simulink model "SF051A_SnsrOffsLrng"  (R2013b)
settings: Solver=FixedStepDiscrete  SolverMode=SingleTasking  StartTime=0.0  StopTime=1  FixedStep=0.002  RelTol=1e-3
values from neighbouring files (symbols this model uses):
  ARCHGLBPRM_10MILLISEC_SEC_F32 = DataDict.Constant    [SF051A_SnsrOffsLrng_DataDict.m]
  ARCHGLBPRM_2MILLISEC_SEC_F32 = DataDict.Constant    [SF051A_SnsrOffsLrng_DataDict.m]
  ARCHGLBPRM_2PI_ULS_F32 = DataDict.Constant    [SF051A_SnsrOffsLrng_DataDict.m]
  ARCHGLBPRM_FLOATZEROTHD_ULS_F32 = DataDict.Constant    [SF051A_SnsrOffsLrng_DataDict.m]
  ARCHGLBPRM_PIOVER180_ULS_F32 = DataDict.Constant    [SF051A_SnsrOffsLrng_DataDict.m]
  CNV100MICROSECTOSEC_SECPERCNT_F32 = DataDict.Constant    [SF051A_SnsrOffsLrng_DataDict.m]
  COVRAMTRXNIT_ULS_F32 = DataDict.Constant    [SF051A_SnsrOffsLrng_DataDict.m]
  HWAGHILIM_HWDEG_F32 = DataDict.Constant    [SF051A_SnsrOffsLrng_DataDict.m]
  HWAUTHYTHD_ULS_F32 = DataDict.Constant    [SF051A_SnsrOffsLrng_DataDict.m]
  HWTQLRNGSTSLRND_CNT_U08 = DataDict.Constant    [SF051A_SnsrOffsLrng_DataDict.m]
  HWTQLRNGSTSNEGOFFS_CNT_U08 = DataDict.Constant    [SF051A_SnsrOffsLrng_DataDict.m]
  HWTQLRNGSTSNOTLRND_CNT_U08 = DataDict.Constant    [SF051A_SnsrOffsLrng_DataDict.m]
  HWTQLRNGSTSPOSOFFS_CNT_U08 = DataDict.Constant    [SF051A_SnsrOffsLrng_DataDict.m]
  HWTQLRNGSTSZEROOFFS_CNT_U08 = DataDict.Constant    [SF051A_SnsrOffsLrng_DataDict.m]
  IDYMTRX_ULS_F32 = DataDict.Constant    [SF051A_SnsrOffsLrng_DataDict.m]
  IVS10MS_ULSPERSEC_F32 = DataDict.Constant    [SF051A_SnsrOffsLrng_DataDict.m]
  LRNGFILTICON_ULS_F32 = DataDict.Constant    [SF051A_SnsrOffsLrng_DataDict.m]
  ONE_ULS_F32 = DataDict.Constant    [SF051A_SnsrOffsLrng_DataDict.m]
  SnsrOffsLrnd = DataDict.NVM    [SF051A_SnsrOffsLrng_DataDict.m]
  SnsrOffsLrngFctEna = DataDict.Calibration    [SF051A_SnsrOffsLrng_DataDict.m]
  SnsrOffsLrngHwAgLrngDrvgDstThd = DataDict.Calibration    [SF051A_SnsrOffsLrng_DataDict.m]
  SnsrOffsLrngHwAgLrngEna = DataDict.Calibration    [SF051A_SnsrOffsLrng_DataDict.m]
  SnsrOffsLrngHwAgLrngHwVelThd = DataDict.Calibration    [SF051A_SnsrOffsLrng_DataDict.m]
  SnsrOffsLrngHwAgLrngSysTqThd = DataDict.Calibration    [SF051A_SnsrOffsLrng_DataDict.m]
  SnsrOffsLrngHwAgLrngSysTqThdMed = DataDict.Calibration    [SF051A_SnsrOffsLrng_DataDict.m]
  SnsrOffsLrngHwAgLrngSysTqThdTrustd = DataDict.Calibration    [SF051A_SnsrOffsLrng_DataDict.m]
  SnsrOffsLrngHwAgLrngSysTqThdWide = DataDict.Calibration    [SF051A_SnsrOffsLrng_DataDict.m]
  SnsrOffsLrngHwAgLrngTi = DataDict.Calibration    [SF051A_SnsrOffsLrng_DataDict.m]
  SnsrOffsLrngHwAgLrngVehSpdThd = DataDict.Calibration    [SF051A_SnsrOffsLrng_DataDict.m]
  SnsrOffsLrngHwAgLrngYawOffsDbnd = DataDict.Calibration    [SF051A_SnsrOffsLrng_DataDict.m]
  SnsrOffsLrngHwAgLrngYawRateThd = DataDict.Calibration    [SF051A_SnsrOffsLrng_DataDict.m]
  SnsrOffsLrngHwAgOffsLim = DataDict.Calibration    [SF051A_SnsrOffsLrng_DataDict.m]
  SnsrOffsLrngHwTqLrngEna = DataDict.Calibration    [SF051A_SnsrOffsLrng_DataDict.m]
  SnsrOffsLrngHwTqLrngEnaTiThd = DataDict.Calibration    [SF051A_SnsrOffsLrng_DataDict.m]
  SnsrOffsLrngHwTqLrngHwAgDbnd = DataDict.Calibration    [SF051A_SnsrOffsLrng_DataDict.m]
  SnsrOffsLrngHwTqLrngHwAgThd = DataDict.Calibration    [SF051A_SnsrOffsLrng_DataDict.m]
  SnsrOffsLrngHwTqLrngHwTqThd = DataDict.Calibration    [SF051A_SnsrOffsLrng_DataDict.m]
  SnsrOffsLrngHwTqLrngHwTqZeroOffsThd = DataDict.Calibration    [SF051A_SnsrOffsLrng_DataDict.m]
  SnsrOffsLrngHwTqLrngHwVelThd = DataDict.Calibration    [SF051A_SnsrOffsLrng_DataDict.m]
  SnsrOffsLrngHwTqLrngMeasTi = DataDict.Calibration    [SF051A_SnsrOffsLrng_DataDict.m]
  SnsrOffsLrngHwTqLrngMeasTiScar = DataDict.Calibration    [SF051A_SnsrOffsLrng_DataDict.m]
  SnsrOffsLrngHwTqLrngSampleImbThd1 = DataDict.Calibration    [SF051A_SnsrOffsLrng_DataDict.m]
  SnsrOffsLrngHwTqLrngSampleImbThd2 = DataDict.Calibration    [SF051A_SnsrOffsLrng_DataDict.m]
  SnsrOffsLrngHwTqLrngSampleThd1 = DataDict.Calibration    [SF051A_SnsrOffsLrng_DataDict.m]
  SnsrOffsLrngHwTqLrngSampleThd2 = DataDict.Calibration    [SF051A_SnsrOffsLrng_DataDict.m]
  SnsrOffsLrngHwTqLrngTiWghtCoeff = DataDict.Calibration    [SF051A_SnsrOffsLrng_DataDict.m]
  SnsrOffsLrngHwTqLrngVehSpdThd = DataDict.Calibration    [SF051A_SnsrOffsLrng_DataDict.m]
  SnsrOffsLrngHwTqOffsLim = DataDict.Calibration    [SF051A_SnsrOffsLrng_DataDict.m]
  SnsrOffsLrngSampleCntForHwTqLrngRst = DataDict.Calibration    [SF051A_SnsrOffsLrng_DataDict.m]
  SnsrOffsLrngTqInpDetnPwrEstimnThd = DataDict.Calibration    [SF051A_SnsrOffsLrng_DataDict.m]
  SnsrOffsLrngTqInpDetnSinGenrAmp = DataDict.Calibration    [SF051A_SnsrOffsLrng_DataDict.m]
  SnsrOffsLrngTqInpDetnSinGenrFrq = DataDict.Calibration    [SF051A_SnsrOffsLrng_DataDict.m]
  SnsrOffsLrngTqInpDetnStg1FilGain = DataDict.Calibration    [SF051A_SnsrOffsLrng_DataDict.m]
  SnsrOffsLrngTqInpDetnStg1WinSize = DataDict.Calibration    [SF051A_SnsrOffsLrng_DataDict.m]
  SnsrOffsLrngTqInpDetnStg2FilGainCen = DataDict.Calibration    [SF051A_SnsrOffsLrng_DataDict.m]
  SnsrOffsLrngTqInpDetnStg2FilGainDwn = DataDict.Calibration    [SF051A_SnsrOffsLrng_DataDict.m]
  SnsrOffsLrngTqInpDetnStg2FilGainUp = DataDict.Calibration    [SF051A_SnsrOffsLrng_DataDict.m]
  SnsrOffsLrngTqInpDetnStg2WinSize = DataDict.Calibration    [SF051A_SnsrOffsLrng_DataDict.m]
  SnsrOffsLrngYawLrngEna = DataDict.Calibration    [SF051A_SnsrOffsLrng_DataDict.m]
  SnsrOffsLrngYawLrngHwAgThd = DataDict.Calibration    [SF051A_SnsrOffsLrng_DataDict.m]
  SnsrOffsLrngYawLrngTi = DataDict.Calibration    [SF051A_SnsrOffsLrng_DataDict.m]
  SnsrOffsLrngYawLrngYawAThd = DataDict.Calibration    [SF051A_SnsrOffsLrng_DataDict.m]
  SnsrOffsLrngYawOffsFrshTiThd = DataDict.Calibration    [SF051A_SnsrOffsLrng_DataDict.m]
  SnsrOffsLrngYawRateOffsLim = DataDict.Calibration    [SF051A_SnsrOffsLrng_DataDict.m]
  SPDCNVN_MTRPERSECPERKPH_F32 = DataDict.Constant    [SF051A_SnsrOffsLrng_DataDict.m]
  SysGlbPrmSysTqRat = DataDict.ImprtdCal    [SF051A_SnsrOffsLrng_DataDict.m]
  TISTEP10MS_MINS_F32 = DataDict.Constant    [SF051A_SnsrOffsLrng_DataDict.m]
  TQINPDETNLOGGAIN_ULS_F32 = DataDict.Constant    [SF051A_SnsrOffsLrng_DataDict.m]
  YAWELPDTIHILIM_MINS_F32 = DataDict.Constant    [SF051A_SnsrOffsLrng_DataDict.m]
  YAWRATENOISE_VEHDEGPERSEC_F32 = DataDict.Constant    [SF051A_SnsrOffsLrng_DataDict.m]
  ZERO_ULS_F32 = DataDict.Constant    [SF051A_SnsrOffsLrng_DataDict.m]
  ZEROVECT_ULS_F32 = DataDict.Constant    [SF051A_SnsrOffsLrng_DataDict.m]
undefined symbols (not defined in the file or in its folder): NvmGetErrSts1
libraries: Fil x34, NxtrLim x20, FixdToFloat x17, FloatToFixd x16, simulink x12, NxtrAbslt x12, NxtrNvM x8, NxtrMath x3
(part 1 of 12)
settings Model: PauseTimes=0  Creator=rz6pnb  LastModifiedBy=TZ5743
settings SolverCC: AutoInsertRateTranBlk=on  InsertRTBMode=Always
settings DataIOCC: LimitDataPoints=off  SaveFormat=Structure  ReturnWorkspaceOutputs=on
settings OptimizationCC: BlockReduction=off  InlineParams=on  ZeroExternalMemoryAtStartup=off  ZeroInternalMemoryAtStartup=off  OptimizeModelRefInitCode=on  LifeSpan=1
settings DebuggingCC: SignalInfNanChecking=error  SignalRangeChecking=warning  UnderspecifiedInitializationDetection=Simplified  SolverPrmCheckMsg=error  InheritedTsInSrcMsg=error  DiscreteInheritContinuousMsg=error  SingleTaskRateTransMsg=error  TasksWithSamePriorityMsg=error  SigSpecEnsureSampleTimeMsg=error  CheckMatrixSingularityMsg=error  ParameterUnderflowMsg=error  ParameterPrecisionLossMsg=error  ParameterTunabilityLossMsg=error  FixptConstUnderflowMsg=warning  FixptConstOverflowMsg=warning  VectorMatrixConversionMsg=error  SignalLabelMismatchMsg=error  UnconnectedInputMsg=error  UnconnectedOutputMsg=error  UnconnectedLineMsg=error  SFcnCompatibilityMsg=error  UniqueDataStoreMsg=warning  BusObjectLabelMismatch=error  RootOutportRequireBusObject=error  AssertControl=DisableAll  ModelReferenceIOMsg=error  ModelReferenceVersionMismatchMessage=warning  ModelReferenceIOMismatchMessage=error  ModelReferenceCSMismatchMessage=warning  ModelReferenceDataLoggingMessage=error  StateNameClashWarn=warning  StrictBusMsg=ErrorOnBusTreatedAsVector  NonBusSignalsTreatedAsBus=error  SFUnexpectedBacktrackingDiag=error  SFInvalidInputDataAccessInChartInitDiag=error  SFNoUnconditionalDefaultTransitionDiag=error  SFTransitionOutsideNaturalParentDiag=error  SFUnconditionalTransitionShadowingDiag=error  SFUndirectedBroadcastEventsDiag=error
settings ModelReferenceCC: ModelReferenceNumInstancesAllowed=Single
settings RTWCC: SystemTargetFile=autosar.tlc  GenCodeOnly=on  TemplateMakefile=ert_default_tmf  Description=AUTOSAR  GenerateReport=on  ProcessScript=autosar_make_rtw_hook  LaunchReport=on
settings CodeAppCC: GenerateComments=off  IgnoreCustomStorageClasses=off  CustomSymbolStrType=$N$R$M  CustomSymbolStrBlkIO=$N$M  SimulinkBlockComments=off
settings STFCustomTargetCC: ParMdlRefBuildCompliant=on  CompOptLevelCompliant=on  IncludeMdlTerminateFcn=off  CombineOutputUpdateFcns=on  SuppressErrorStatus=on  ERTFirstTimeCompliant=on  ERTCustomFileBanners=on  SupportNonFinite=off  SupportComplex=off  SupportContinuousTime=off  SupportNonInlinedSFcns=off  MATLABClassNameForMDSCustomization=Simulink.SoftwareTarget.ERTCustomization  AutosarCompliant=on  GRTInterface=off  SystemTargetFile=autosar.tlc
settings ERTTargetCC: CodeReplacementLibrary=ANSI_C  ConcurrentExecutionCompliant=off  IncludeMdlTerminateFcn=off  SuppressErrorStatus=on  SupportNonFinite=off  SupportComplex=off  ModelStepFunctionPrototypeControlCompliant=off  CPPClassGenCompliant=off  AutosarCompliant=on  InlinedParameterPlacement=NonHierarchical  ERTCustomFileTemplate=example_file_process.tlc  EnableUserReplacementTypes=on

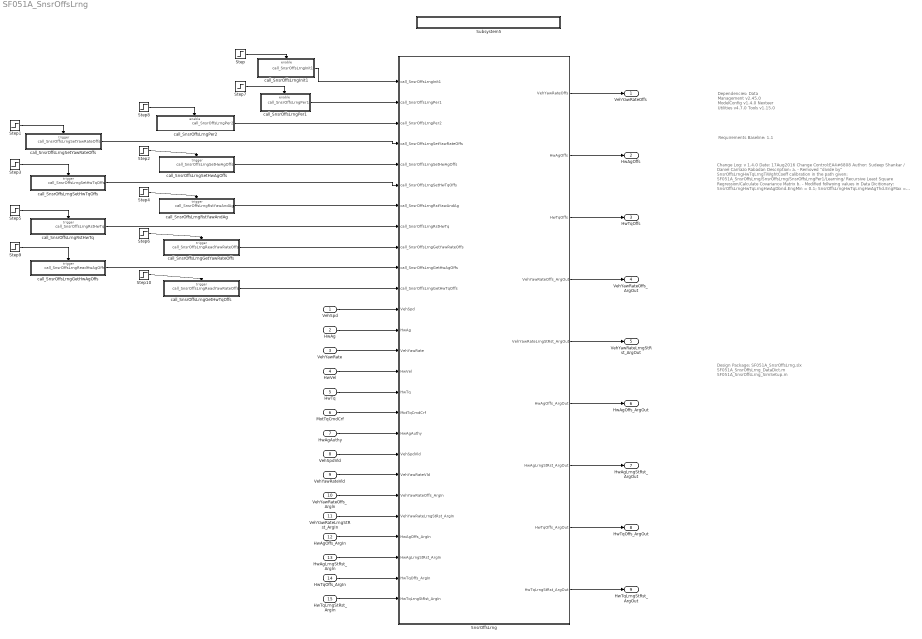
== system SF051A_SnsrOffsLrng ==
  note: Requirements Baseline: 1.1
  note: Change Log:
      |
      | v 1.4.0
      | Date: 17Aug2016
      | Change Control:EA4#6808
      | Author: Sudeep Shankar / Daniel Carriazo Rabadan
      | Description:
      | a. - Removed "divide by" SnsrOffsLrngHwTqLrngTiWghtCoeff calibration
      | in the path given:
      |  SF051A_SnsrOffsLrng/SnsrOffsLrng/SnsrOffsLrngPer1/Learning/
      | Recursive Least Square Regression/Calculate Covariance Matrix
      |
      | b. - Modified follwoing values in Data Dicitionary:
      | SnsrOffsLrngHwTqLrngHwAgDbnd.EngMin = 0.1;
      | SnsrOffsLrngHwTqLrngHwAgThd.EngMax = 180;
      | SnsrOffsLrngHwTqLrngHwTqThd.EngMax = 3;
      | SnsrOffsLrngHwTqLrngMeasTiScar.EngMin = 1;
      | SnsrOffsLrngHwTqLrngSampleThd1.EngMin = 1;
      | SnsrOffsLrngHwTqLrngSampleThd2.EngMin = 1;
      | SnsrOffsLrngTqInpDetnStg2WinSize.EngMax = 65463;
      |
      | c. - Added logic to reset the learning calculations when HwAg mesarured
      | count exceeds calibration value.
      | - Added calibration  SnsrOffsLrngSampleCntForHwTqLrngRst in Data Dictionary
      |
      |
      | v 1.3.1
      | Date: 6Jun2016
      | Change Control:EA4#5906
      | Author: Sudeep Shankar
      | Description:
      | -  Created links to DOORS requirements
      |
      | v 1.3.0
      | Date: 9May2016
      | Change Control:EA4#5625
      | Author: Sudeep Shankar
      | Description:
      | - Eng.Min value of "SnsrOffsLrngHwTqLrngMeasTi" changed
      | from 0 to 0.01 in Data Dictionary.
      |
      | v 1.2.0
      | Date: 3Mar2016
      | Change Control:EA4#4004
      | Author: Sudeep Shankar
      | Description:
      | Included 3 Read Server Runnables
      |
      | v 1.1.0
      | Date: 25Feb2016
      | Change Control:EA4#4004
      | Author: Sudeep Shankar
      | Description:
      | 1. Removed Trans1 function and replaced2.
      | 2. write to data store block 'SetRamBlkSts' is
      | replaced by NVM block 'Set Ram Block Status' in
      | following path:
      | SnsrOffsLrng/SnsrOffsLrngInit1/NVM Management/Not Enabled
      | SnsrOffsLrng/SnsrOffsLrngInit1/NVM Management/Data Valid
      | SnsrOffsLrng/SnsrOffsLrngInit1/NVM Management/Data Invalid
      | SnsrOffsLrng/SetYawRateOffs
      | SnsrOffsLrng/SetHwTqOffs
      | SnsrOffsLrng/SetHwAgOffs
      | SnsrOffsLrng/RstYawAndAg
      | SnsrOffsLrng/RstHwTq
      | 3. Removed 'Set Ram Block Status' to False in the below path:
      | SnsrOffsLrng/SnsrOffsLrngInit1/NVM Management/Not Enabled
      |
      | v 1.0.0
      | Date: 20Jan2016
      | Change Control:EA4#3125
      | Author:Praveen Devaraj(KPIT)
      | Description:
      | Initial EA4 Version from EA3 v2.0.0
  note: Dependencies:
      |    Data Management v2.45.0
      |    ModelConfig v1.4.0
      |    Nexteer Utilities v4.7.0
      |    Tools v1.15.0
  note: Design Package:
      | SF051A_SnsrOffsLrng.slx
      | SF051A_SnsrOffsLrng_DataDict.m
      | SF051A_SnsrOffsLrng_SimSetup.m
  VehSpd : Inport
  HwAg : Inport  Port=2
  VehYawRate : Inport  Port=3
  HwVel : Inport  Port=4
  HwTq : Inport  Port=5
  MotTqCmdCrf : Inport  Port=6
  HwAgAuthy : Inport  Port=7
  VehSpdVld : Inport  Port=8
  VehYawRateVld : Inport  Port=9
  VehYawRateOffs_Argln : Inport  Port=10
  VehYawRateLrngStRst_ArgIn : Inport  Port=11
  HwAgOffs_ArgIn : Inport  Port=12
  HwAgLrngStRst_ArgIn : Inport  Port=13
  HwTqOffs_ArgIn : Inport  Port=14
  HwTqLrngStRst_ArgIn : Inport  Port=15
  " call_SnsrOffsLrngGetHwAgOffs" : Subsystem  TreatAsAtomicUnit=on
  " call_SnsrOffsLrngGetHwTqOffs" : Subsystem  TreatAsAtomicUnit=on
  " call_SnsrOffsLrngGetYawRateOffs" : Subsystem  TreatAsAtomicUnit=on
  " call_SnsrOffsLrngRstHwTq" : Subsystem  TreatAsAtomicUnit=on
  " call_SnsrOffsLrngRstYawAndAg" : Subsystem  TreatAsAtomicUnit=on
  " call_SnsrOffsLrngSetHwAgOffs" : Subsystem  TreatAsAtomicUnit=on
  " call_SnsrOffsLrngSetHwTqOffs" : Subsystem  TreatAsAtomicUnit=on
  " call_SnsrOffsLrngSetYawRateOffs" : Subsystem  TreatAsAtomicUnit=on
  SnsrOffsLrng : Subsystem
  Step : Step  Time=0.0005  Before=1  After=0  SampleTime=0
  Step{1..6,9..10} (8 alike) : Step  Time=0.3  SampleTime=0
  Step7 : Step  Time=0.002  SampleTime=0
  Step8 : Step  Time=0.0005  SampleTime=0
  Subsystem5 : Subsystem  Description=|  mask(Copyright Information){none=on}
      | Copyright info block.                                               
      |                                                                     
      | Place copyright information at the top of every subsystem in design.
      mask prompts: none "No parameters"
      mask help: Place copyright information at the top of every subsystem in design.
      mask Display:
      | NxtrConf = 'Nexteer Confidential';
      | 
      | sys = bdroot; %handle for the current model ("system")
      | first = get_param(sys,'Created');
      | first = first(end-3:end);  %year is last four digits
      | 
      | last = get_param(sys,'LastModifiedDate');
      | if isempty(last)
      |     last = datestr(now,'yyyy');
      | else
      |     last = last(end-3:end);
      | end
      | 
      | if strcmp(first,last)
      |     fprintf('%s -- Copyright %s Nexteer',NxtrConf,first)
      | else
      |     fprintf('%s -- %s%s- %s Nexteer',NxtrConf,char(169),first,last)
      | end
  call_SnsrOffsLrngInit1 : Subsystem  TreatAsAtomicUnit=on
  call_SnsrOffsLrngPer1 : Subsystem  TreatAsAtomicUnit=on
  call_SnsrOffsLrngPer2 : Subsystem  TreatAsAtomicUnit=on
  VehYawRateOffs : Outport
  HwAgOffs : Outport  Port=2
  HwTqOffs : Outport  Port=3
  VehYawRateOffs_ArgOut : Outport  Port=4
  VehYawRateLrngStRst_ArgOut : Outport  Port=5
  HwAgOffs_ArgOut : Outport  Port=6
  HwAgLrngStRst_ArgOut : Outport  Port=7
  HwTqOffs_ArgOut : Outport  Port=8
  HwTqLrngStRst_ArgOut : Outport  Port=9
  wires:
  call_SnsrOffsLrngPer1/1(call_SnsrOffsLrngPer1) -> SnsrOffsLrng/2(call_SnsrOffsLrngPer1)
  call_SnsrOffsLrngInit1/1(call_SnsrOffsLrngInit1) -> SnsrOffsLrng/1(call_SnsrOffsLrngInit1)
  SnsrOffsLrng/1(VehYawRateOffs) -> VehYawRateOffs/1
  Step/1 -> call_SnsrOffsLrngInit1/Enable
  " call_SnsrOffsLrngSetHwTqOffs"/1(call_SnsrOffsLrngSetHwTqOffs) -> SnsrOffsLrng/6(call_SnsrOffsLrngSetHwTqOffs)
  " call_SnsrOffsLrngSetHwAgOffs"/1(call_SnsrOffsLrngSetHwAgOffs) -> SnsrOffsLrng/5(call_SnsrOffsLrngSetHwAgOffs)
  " call_SnsrOffsLrngRstYawAndAg"/1(call_SnsrOffsLrngRstYawAndAg) -> SnsrOffsLrng/7(call_SnsrOffsLrngRstYawAndAg)
  call_SnsrOffsLrngPer2/1(call_SnsrOffsLrngPer2) -> SnsrOffsLrng/3(call_SnsrOffsLrngPer2)
  SnsrOffsLrng/2(HwAgOffs) -> HwAgOffs/1
  SnsrOffsLrng/3(HwTqOffs) -> HwTqOffs/1
  " call_SnsrOffsLrngRstHwTq"/1(call_SnsrOffsLrngRstHwTq) -> SnsrOffsLrng/8(call_SnsrOffsLrngRstHwTq)
  " call_SnsrOffsLrngSetYawRateOffs"/1(call_SnsrOffsLrngSetYawRateOffs) -> SnsrOffsLrng/4(call_SnsrOffsLrngSetYawRateOffs)
  HwAg/1 -> SnsrOffsLrng/13(HwAg)
  HwVel/1 -> SnsrOffsLrng/15(HwVel)
  VehSpd/1 -> SnsrOffsLrng/12(VehSpd)
  HwTqOffs_ArgIn/1 -> SnsrOffsLrng/25(HwTqOffs_ArgIn)
  VehYawRate/1 -> SnsrOffsLrng/14(VehYawRate)
  HwAgOffs_ArgIn/1 -> SnsrOffsLrng/23(HwAgOffs_ArgIn)
  HwAgLrngStRst_ArgIn/1 -> SnsrOffsLrng/24(HwAgLrngStRst_ArgIn)
  HwTq/1 -> SnsrOffsLrng/16(HwTq)
  MotTqCmdCrf/1 -> SnsrOffsLrng/17(MotTqCmdCrf)
  HwAgAuthy/1 -> SnsrOffsLrng/18(HwAgAuthy)
  VehSpdVld/1 -> SnsrOffsLrng/19(VehSpdVld)
  VehYawRateVld/1 -> SnsrOffsLrng/20(VehYawRateVld)
  VehYawRateOffs_Argln/1 -> SnsrOffsLrng/21(VehYawRateOffs_ArgIn)
  VehYawRateLrngStRst_ArgIn/1 -> SnsrOffsLrng/22(VehYawRateLrngStRst_ArgIn)
  HwTqLrngStRst_ArgIn/1 -> SnsrOffsLrng/26(HwTqLrngStRst_ArgIn)
  Step7/1 -> call_SnsrOffsLrngPer1/Enable
  Step8/1 -> call_SnsrOffsLrngPer2/Enable
  Step1/1 -> " call_SnsrOffsLrngSetYawRateOffs"/Trigger
  Step2/1 -> " call_SnsrOffsLrngSetHwAgOffs"/Trigger
  Step3/1 -> " call_SnsrOffsLrngSetHwTqOffs"/Trigger
  Step4/1 -> " call_SnsrOffsLrngRstYawAndAg"/Trigger
  Step5/1 -> " call_SnsrOffsLrngRstHwTq"/Trigger
  SnsrOffsLrng/4(VehYawRateOffs_ArgOut) -> VehYawRateOffs_ArgOut/1
  SnsrOffsLrng/5(VehYawRateLrngStRst_ArgOut) -> VehYawRateLrngStRst_ArgOut/1
  SnsrOffsLrng/6(HwAgOffs_ArgOut) -> HwAgOffs_ArgOut/1
  SnsrOffsLrng/7(HwAgLrngStRst_ArgOut) -> HwAgLrngStRst_ArgOut/1
  SnsrOffsLrng/8(HwTqOffs_ArgOut) -> HwTqOffs_ArgOut/1
  SnsrOffsLrng/9(HwTqLrngStRst_ArgOut) -> HwTqLrngStRst_ArgOut/1
  Step6/1 -> " call_SnsrOffsLrngGetYawRateOffs"/Trigger
  " call_SnsrOffsLrngGetYawRateOffs"/1(call_SnsrOffsLrngReadYawRateOffs) -> SnsrOffsLrng/9(call_SnsrOffsLrngGetYawRateOffs)
  " call_SnsrOffsLrngGetHwAgOffs"/1(call_SnsrOffsLrngReadHwAgOffs) -> SnsrOffsLrng/10(call_SnsrOffsLrngGetHwAgOffs)
  Step9/1 -> " call_SnsrOffsLrngGetHwAgOffs"/Trigger
  " call_SnsrOffsLrngGetHwTqOffs"/1(call_SnsrOffsLrngReadYawRateOffs) -> SnsrOffsLrng/11(call_SnsrOffsLrngGetHwTqOffs)
  Step10/1 -> " call_SnsrOffsLrngGetHwTqOffs"/Trigger

== system SF051A_SnsrOffsLrng/ call_SnsrOffsLrngGetHwAgOffs ==
  Trigger : TriggerPort  PortDimensions=1
  FunctionCallGenerator : simulink/Ports & Subsystems/Function-Call Generator  sample_time=-1  numberOfIterations=1
  Subsystem5 : Subsystem  Description=|  mask(Copyright Information){none=on}
      | Copyright info block.                                               
      |                                                                     
      | Place copyright information at the top of every subsystem in design.
      mask prompts: none "No parameters"
      mask help: Place copyright information at the top of every subsystem in design.
      mask Display:
      | NxtrConf = 'Nexteer Confidential';
      | 
      | sys = bdroot; %handle for the current model ("system")
      | first = get_param(sys,'Created');
      | first = first(end-3:end);  %year is last four digits
      | 
      | last = get_param(sys,'LastModifiedDate');
      | if isempty(last)
      |     last = datestr(now,'yyyy');
      | else
      |     last = last(end-3:end);
      | end
      | 
      | if strcmp(first,last)
      |     fprintf('%s -- Copyright %s Nexteer',NxtrConf,first)
      | else
      |     fprintf('%s -- %s%s- %s Nexteer',NxtrConf,char(169),first,last)
      | end
  call_SnsrOffsLrngReadHwAgOffs : Outport
  wires:
  FunctionCallGenerator/1 -> call_SnsrOffsLrngReadHwAgOffs/1

== system SF051A_SnsrOffsLrng/ call_SnsrOffsLrngGetHwTqOffs ==
  Trigger : TriggerPort  PortDimensions=1
  FunctionCallGenerator : simulink/Ports & Subsystems/Function-Call Generator  sample_time=-1  numberOfIterations=1
  Subsystem5 : Subsystem  Description=|  mask(Copyright Information){none=on}
      | Copyright info block.                                               
      |                                                                     
      | Place copyright information at the top of every subsystem in design.
      mask prompts: none "No parameters"
      mask help: Place copyright information at the top of every subsystem in design.
      mask Display:
      | NxtrConf = 'Nexteer Confidential';
      | 
      | sys = bdroot; %handle for the current model ("system")
      | first = get_param(sys,'Created');
      | first = first(end-3:end);  %year is last four digits
      | 
      | last = get_param(sys,'LastModifiedDate');
      | if isempty(last)
      |     last = datestr(now,'yyyy');
      | else
      |     last = last(end-3:end);
      | end
      | 
      | if strcmp(first,last)
      |     fprintf('%s -- Copyright %s Nexteer',NxtrConf,first)
      | else
      |     fprintf('%s -- %s%s- %s Nexteer',NxtrConf,char(169),first,last)
      | end
  call_SnsrOffsLrngReadYawRateOffs : Outport
  wires:
  FunctionCallGenerator/1 -> call_SnsrOffsLrngReadYawRateOffs/1

== system SF051A_SnsrOffsLrng/ call_SnsrOffsLrngGetYawRateOffs ==
  Trigger : TriggerPort  PortDimensions=1
  FunctionCallGenerator : simulink/Ports & Subsystems/Function-Call Generator  sample_time=-1  numberOfIterations=1
  Subsystem5 : Subsystem  Description=|  mask(Copyright Information){none=on}
      | Copyright info block.                                               
      |                                                                     
      | Place copyright information at the top of every subsystem in design.
      mask prompts: none "No parameters"
      mask help: Place copyright information at the top of every subsystem in design.
      mask Display:
      | NxtrConf = 'Nexteer Confidential';
      | 
      | sys = bdroot; %handle for the current model ("system")
      | first = get_param(sys,'Created');
      | first = first(end-3:end);  %year is last four digits
      | 
      | last = get_param(sys,'LastModifiedDate');
      | if isempty(last)
      |     last = datestr(now,'yyyy');
      | else
      |     last = last(end-3:end);
      | end
      | 
      | if strcmp(first,last)
      |     fprintf('%s -- Copyright %s Nexteer',NxtrConf,first)
      | else
      |     fprintf('%s -- %s%s- %s Nexteer',NxtrConf,char(169),first,last)
      | end
  call_SnsrOffsLrngReadYawRateOffs : Outport
  wires:
  FunctionCallGenerator/1 -> call_SnsrOffsLrngReadYawRateOffs/1

== system SF051A_SnsrOffsLrng/ call_SnsrOffsLrngRstHwTq ==
  Trigger : TriggerPort  PortDimensions=1
  FunctionCallGenerator : simulink/Ports & Subsystems/Function-Call Generator  sample_time=-1  numberOfIterations=1
  Subsystem5 : Subsystem  Description=|  mask(Copyright Information){none=on}
      | Copyright info block.                                               
      |                                                                     
      | Place copyright information at the top of every subsystem in design.
      mask prompts: none "No parameters"
      mask help: Place copyright information at the top of every subsystem in design.
      mask Display:
      | NxtrConf = 'Nexteer Confidential';
      | 
      | sys = bdroot; %handle for the current model ("system")
      | first = get_param(sys,'Created');
      | first = first(end-3:end);  %year is last four digits
      | 
      | last = get_param(sys,'LastModifiedDate');
      | if isempty(last)
      |     last = datestr(now,'yyyy');
      | else
      |     last = last(end-3:end);
      | end
      | 
      | if strcmp(first,last)
      |     fprintf('%s -- Copyright %s Nexteer',NxtrConf,first)
      | else
      |     fprintf('%s -- %s%s- %s Nexteer',NxtrConf,char(169),first,last)
      | end
  call_SnsrOffsLrngRstHwTq : Outport
  wires:
  FunctionCallGenerator/1 -> call_SnsrOffsLrngRstHwTq/1

== system SF051A_SnsrOffsLrng/ call_SnsrOffsLrngRstYawAndAg ==
  Trigger : TriggerPort  PortDimensions=1
  FunctionCallGenerator : simulink/Ports & Subsystems/Function-Call Generator  sample_time=-1  numberOfIterations=1
  Subsystem5 : Subsystem  Description=|  mask(Copyright Information){none=on}
      | Copyright info block.                                               
      |                                                                     
      | Place copyright information at the top of every subsystem in design.
      mask prompts: none "No parameters"
      mask help: Place copyright information at the top of every subsystem in design.
      mask Display:
      | NxtrConf = 'Nexteer Confidential';
      | 
      | sys = bdroot; %handle for the current model ("system")
      | first = get_param(sys,'Created');
      | first = first(end-3:end);  %year is last four digits
      | 
      | last = get_param(sys,'LastModifiedDate');
      | if isempty(last)
      |     last = datestr(now,'yyyy');
      | else
      |     last = last(end-3:end);
      | end
      | 
      | if strcmp(first,last)
      |     fprintf('%s -- Copyright %s Nexteer',NxtrConf,first)
      | else
      |     fprintf('%s -- %s%s- %s Nexteer',NxtrConf,char(169),first,last)
      | end
  call_SnsrOffsLrngRstYawAndAg : Outport
  wires:
  FunctionCallGenerator/1 -> call_SnsrOffsLrngRstYawAndAg/1

== system SF051A_SnsrOffsLrng/ call_SnsrOffsLrngSetHwAgOffs ==
  Trigger : TriggerPort  PortDimensions=1
  FunctionCallGenerator : simulink/Ports & Subsystems/Function-Call Generator  sample_time=-1  numberOfIterations=1
  Subsystem5 : Subsystem  Description=|  mask(Copyright Information){none=on}
      | Copyright info block.                                               
      |                                                                     
      | Place copyright information at the top of every subsystem in design.
      mask prompts: none "No parameters"
      mask help: Place copyright information at the top of every subsystem in design.
      mask Display:
      | NxtrConf = 'Nexteer Confidential';
      | 
      | sys = bdroot; %handle for the current model ("system")
      | first = get_param(sys,'Created');
      | first = first(end-3:end);  %year is last four digits
      | 
      | last = get_param(sys,'LastModifiedDate');
      | if isempty(last)
      |     last = datestr(now,'yyyy');
      | else
      |     last = last(end-3:end);
      | end
      | 
      | if strcmp(first,last)
      |     fprintf('%s -- Copyright %s Nexteer',NxtrConf,first)
      | else
      |     fprintf('%s -- %s%s- %s Nexteer',NxtrConf,char(169),first,last)
      | end
  call_SnsrOffsLrngSetHwAgOffs : Outport
  wires:
  FunctionCallGenerator/1 -> call_SnsrOffsLrngSetHwAgOffs/1

== system SF051A_SnsrOffsLrng/ call_SnsrOffsLrngSetHwTqOffs ==
  Trigger : TriggerPort  PortDimensions=1
  FunctionCallGenerator : simulink/Ports & Subsystems/Function-Call Generator  sample_time=-1  numberOfIterations=1
  Subsystem5 : Subsystem  Description=|  mask(Copyright Information){none=on}
      | Copyright info block.                                               
      |                                                                     
      | Place copyright information at the top of every subsystem in design.
      mask prompts: none "No parameters"
      mask help: Place copyright information at the top of every subsystem in design.
      mask Display:
      | NxtrConf = 'Nexteer Confidential';
      | 
      | sys = bdroot; %handle for the current model ("system")
      | first = get_param(sys,'Created');
      | first = first(end-3:end);  %year is last four digits
      | 
      | last = get_param(sys,'LastModifiedDate');
      | if isempty(last)
      |     last = datestr(now,'yyyy');
      | else
      |     last = last(end-3:end);
      | end
      | 
      | if strcmp(first,last)
      |     fprintf('%s -- Copyright %s Nexteer',NxtrConf,first)
      | else
      |     fprintf('%s -- %s%s- %s Nexteer',NxtrConf,char(169),first,last)
      | end
  call_SnsrOffsLrngSetHwTqOffs : Outport
  wires:
  FunctionCallGenerator/1 -> call_SnsrOffsLrngSetHwTqOffs/1

== system SF051A_SnsrOffsLrng/ call_SnsrOffsLrngSetYawRateOffs ==
  Trigger : TriggerPort  PortDimensions=1
  FunctionCallGenerator : simulink/Ports & Subsystems/Function-Call Generator  sample_time=-1  numberOfIterations=1
  Subsystem5 : Subsystem  Description=|  mask(Copyright Information){none=on}
      | Copyright info block.                                               
      |                                                                     
      | Place copyright information at the top of every subsystem in design.
      mask prompts: none "No parameters"
      mask help: Place copyright information at the top of every subsystem in design.
      mask Display:
      | NxtrConf = 'Nexteer Confidential';
      | 
      | sys = bdroot; %handle for the current model ("system")
      | first = get_param(sys,'Created');
      | first = first(end-3:end);  %year is last four digits
      | 
      | last = get_param(sys,'LastModifiedDate');
      | if isempty(last)
      |     last = datestr(now,'yyyy');
      | else
      |     last = last(end-3:end);
      | end
      | 
      | if strcmp(first,last)
      |     fprintf('%s -- Copyright %s Nexteer',NxtrConf,first)
      | else
      |     fprintf('%s -- %s%s- %s Nexteer',NxtrConf,char(169),first,last)
      | end
  call_SnsrOffsLrngSetYawRateOffs : Outport
  wires:
  FunctionCallGenerator/1 -> call_SnsrOffsLrngSetYawRateOffs/1
